simulink model "Molehill"  (Simulink 8.5)
settings: Solver=ode3  StartTime=0.0  StopTime=inf  FixedStep=0.001  RelTol=1e-3
undefined symbols (not defined in the file or in its folder): seedc, seedn
libraries: slrtlib x7, xpcquanserlib x4
settings Model: Creator=Ninad  LastModifiedBy=Ryan  SimulationMode=external
settings SolverCC: EnableConcurrentExecution=on
settings OptimizationCC: BlockReduction=off  OptimizeBlockIOStorage=off  BufferReuse=off  GlobalBufferReuse=off  ExpressionFolding=off  LocalBlockOutputs=off
settings DebuggingCC: SolverPrmCheckMsg=warning  FcnCallInpInsideContextMsg=UseLocalSettings
settings HardwareCC: ProdIntDivRoundTo=Zero  ProdEndianess=LittleEndian  ProdLongLongMode=on  ProdHWDeviceType=Generic->32-bit x86 compatible
settings RTWCC: SystemTargetFile=slrt.tlc  TemplateMakefile=slrt_default_tmf  Description=Simulink Real-Time  RTWCompilerOptimization=on
settings SimulinkRealTimeCC: GeneratePreprocessorConditionals=Disable all

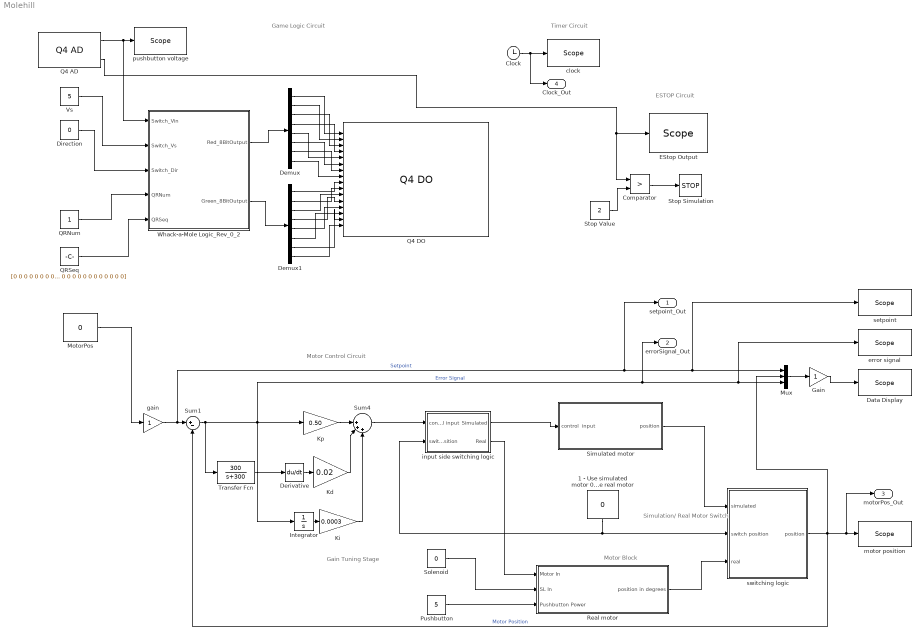
== system Molehill ==
  note: Gain Tuning Stage
  note: Motor Control Circuit
  note: Simulation/
      | Real Motor
      | Switch
  note: Game Logic Circuit
  note: ESTOP Circuit
  note: Timer Circuit
  note: Motor Block
  1 - Use simulated motor 0 - Use real motor : Constant  Value=0
  Clock : Clock
  Comparator : RelationalOperator  Operator=>  OutDataTypeStr=boolean
  Data Display : slrtlib/Displays and Logging/Scope   scopeno=3  scopetype=Target  autostart=on  viewmode=Numerical  formatstr="'Setpoint        %3.2f,Motor Position  %3.2f,Error Signal    %3.2f'"  grid=on  ylimits=[0,170]  nosamples=200  noprepostsamples=0  interleave=10  triggermode=FreeRun  triggersignal=1  trigsignalfromport=off  triggerlevel=0.0  triggerslope=Either  triggerscope=1  triggersample=0  filename=data.dat  mode=Lazy  writesize=512  autorestart=off  dynamicfilemode=off  maxwritefilesize=512*1024^2
  Demux : Demux  Outputs=8
  Demux1 : Demux  Outputs=8
  Derivative : Derivative
  Direction : Constant  Value=0
  "EStop Output " : slrtlib/Displays and Logging/Scope   scopeno=6  scopetype=Target  autostart=on  viewmode=Graphical redraw  formatstr='%15.6f'  grid=on  ylimits=[-6,6]  nosamples=250  noprepostsamples=0  interleave=1  triggermode=FreeRun  triggersignal=1  trigsignalfromport=off  triggerlevel=0.0  triggerslope=Either  triggerscope=1  triggersample=0  filename=data.dat  mode=Lazy  writesize=512  autorestart=off  dynamicfilemode=off  maxwritefilesize=512*1024^2
  Gain : Gain
  Integrator : Integrator
  Kd : Gain  Gain=0.02
  Ki : Gain  Gain=0.0003
  Kp : Gain  Gain=0.50
  MotorPos : Constant  Value=0
  Mux : Mux  Inputs=3
  Pushbutton : Constant  Value=5
  Q4 AD : xpcquanserlib/A//D/Q4 AD  channel=[3 4]  sampleTime=0.001  slot=-1
  "Q4 DO " : xpcquanserlib/Digital Output/Q4 DO   channel=[1 2 3 4 5 6 7 8 9 10 11 12 13 14 15 16]  reset=[1]  initValue=[0 0 0 0 0 0 0 0 0 0 0 0 0 0 0 0]  sampleTime=.001  slot=-1
  QRNum : Constant
  QRSeq : Constant  Value=[0 0 0 0 0 0 0 0 0 0 0 0 0 0 0 0 0 0 0 0]
  Real motor : Subsystem
  Simulated motor : Subsystem
  Solenoid : Constant  Value=0
  Stop Simulation : Stop
  Stop Value : Constant  Value=2
  Sum1 : Sum  Inputs=|+-
  Sum4 : Sum  Inputs=||+++
  Transfer Fcn : TransferFcn  Numerator=[300]  Denominator=[1 300]
  Vs : Constant  Value=5
  Whack-a-Mole Logic_Rev_0_2 : Subsystem  StartFcn=|
      | seedc=seedc+1;
      | seedn=seedn+1;
  clock : slrtlib/Displays and Logging/Scope   scopeno=5  scopetype=Target  autostart=on  viewmode=Numerical  formatstr='%1.3f'  grid=on  ylimits=[-0.2, 1.2]  nosamples=250  noprepostsamples=0  interleave=1  triggermode=FreeRun  triggersignal=1  trigsignalfromport=off  triggerlevel=0.0  triggerslope=Either  triggerscope=1  triggersample=0  filename=data.dat  mode=Lazy  writesize=512  autorestart=off  dynamicfilemode=off  maxwritefilesize=512*1024^2
  error signal : slrtlib/Displays and Logging/Scope   scopeno=2  scopetype=Target  autostart=on  viewmode=Graphical rolling  formatstr='%15.6f'  grid=on  ylimits=[-180,180]  nosamples=500  noprepostsamples=0  interleave=10  triggermode=FreeRun  triggersignal=1  trigsignalfromport=off  triggerlevel=0.0  triggerslope=Either  triggerscope=1  triggersample=0  filename=data.dat  mode=Lazy  writesize=512  autorestart=off  dynamicfilemode=off  maxwritefilesize=512*1024^2
  gain : Gain
  input side switching logic : Subsystem
  motor position : slrtlib/Displays and Logging/Scope   scopeno=7  scopetype=Target  autostart=on  viewmode=Graphical rolling  formatstr='%15.6f'  grid=on  ylimits=[-180,180]  nosamples=500  noprepostsamples=0  interleave=10  triggermode=FreeRun  triggersignal=1  trigsignalfromport=off  triggerlevel=0.0  triggerslope=Either  triggerscope=1  triggersample=0  filename=data.dat  mode=Lazy  writesize=512  autorestart=off  dynamicfilemode=off  maxwritefilesize=512*1024^2
  "pushbutton voltage " : slrtlib/Displays and Logging/Scope   scopeno=4  scopetype=Target  autostart=on  viewmode=Numerical  formatstr='%1.3f'  grid=on  ylimits=[-0.2, 1.2]  nosamples=250  noprepostsamples=0  interleave=1  triggermode=FreeRun  triggersignal=1  trigsignalfromport=off  triggerlevel=0.0  triggerslope=Either  triggerscope=1  triggersample=0  filename=data.dat  mode=Lazy  writesize=512  autorestart=off  dynamicfilemode=off  maxwritefilesize=512*1024^2
  setpoint : slrtlib/Displays and Logging/Scope   scopeno=1  scopetype=Target  autostart=on  viewmode=Graphical rolling  formatstr='%15.6f'  grid=on  ylimits=[-180,180]  nosamples=500  noprepostsamples=0  interleave=10  triggermode=FreeRun  triggersignal=1  trigsignalfromport=off  triggerlevel=0.0  triggerslope=Either  triggerscope=1  triggersample=0  filename=data.dat  mode=Lazy  writesize=512  autorestart=off  dynamicfilemode=off  maxwritefilesize=512*1024^2
  switching logic : Subsystem
  setpoint_Out : Outport
  errorSignal_Out : Outport  Port=2
  motorPos_Out : Outport  Port=3
  Clock_Out : Outport  Port=4
  wires:
  Kp/1 -> Sum4/1
  Kd/1 -> Sum4/2
  Derivative/1 -> Kd/1
  Integrator/1 -> Ki/1
  Ki/1 -> Sum4/3
  gain/1 -> Sum1/1, Mux/1, setpoint/1, setpoint_Out/1  "Setpoint"
  MotorPos/1 -> gain/1
  input side switching logic/1(Simulated) -> Simulated motor/1(control  input)
  input side switching logic/2(Real) -> Real motor/1(Motor In)
  Simulated motor/1(position) -> switching logic/1(simulated)
  Real motor/1(position in degrees) -> switching logic/3(real)
  switching logic/1(position) -> Mux/2, Sum1/2, motor position/1, motorPos_Out/1  "Motor Position"
  Sum4/1 -> input side switching logic/1(control input)
  1 - Use simulated motor 0 - Use real motor/1 -> switching logic/2(switch position), input side switching logic/2(switch  position)
  Gain/1 -> Data Display/1
  Mux/1 -> Gain/1
  Sum1/1 -> Mux/3, error signal/1, errorSignal_Out/1, Kp/1, Integrator/1, Transfer Fcn/1  "Error Signal"
  Comparator/1 -> Stop Simulation/1
  Stop Value/1 -> Comparator/2
  Q4 AD/2 -> Comparator/1, "EStop Output "/1
  Clock/1 -> Clock_Out/1, clock/1
  Whack-a-Mole Logic_Rev_0_2/1(Red_8BitOutput) -> Demux/1
  Whack-a-Mole Logic_Rev_0_2/2(Green_8BitOutput) -> Demux1/1
  Direction/1 -> Whack-a-Mole Logic_Rev_0_2/3(Switch_Dir)
  Vs/1 -> Whack-a-Mole Logic_Rev_0_2/2(Switch_Vs)
  QRNum/1 -> Whack-a-Mole Logic_Rev_0_2/4(QRNum)
  QRSeq/1 -> Whack-a-Mole Logic_Rev_0_2/5(QRSeq)
  Q4 AD/1 -> Whack-a-Mole Logic_Rev_0_2/1(Switch_Vin), "pushbutton voltage "/1
  Demux/8 -> "Q4 DO "/8
  Demux/7 -> "Q4 DO "/7
  Demux/6 -> "Q4 DO "/6
  Demux/5 -> "Q4 DO "/5
  Demux/4 -> "Q4 DO "/4
  Demux/3 -> "Q4 DO "/3
  Demux/2 -> "Q4 DO "/2
  Demux/1 -> "Q4 DO "/1
  Demux1/1 -> "Q4 DO "/9
  Demux1/2 -> "Q4 DO "/10
  Demux1/3 -> "Q4 DO "/11
  Demux1/4 -> "Q4 DO "/12
  Demux1/5 -> "Q4 DO "/13
  Demux1/6 -> "Q4 DO "/14
  Demux1/7 -> "Q4 DO "/15
  Demux1/8 -> "Q4 DO "/16
  Transfer Fcn/1 -> Derivative/1
  Solenoid/1 -> Real motor/2(SL In)
  Pushbutton/1 -> Real motor/3(Pushbutton Power)

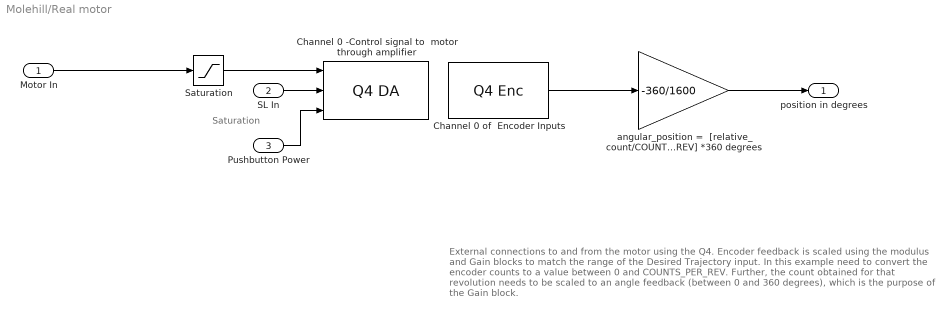
== system Molehill/Real motor ==
  note: Saturation
  note: External connections to and from the motor using the Q4.
      |
      | Encoder feedback is scaled using the modulus and Gain blocks to
      | match the range of the Desired Trajectory input.
      |
      | In this example need to convert the encoder counts to a value between 0 and COUNTS_PER_REV.
      | Further, the count obtained for that revolution needs to be scaled to an angle feedback (between
      | 0 and 360 degrees), which is the purpose of the Gain block.
  Motor In : Inport
  SL In : Inport  Port=2
  Pushbutton Power : Inport  Port=3
  "Channel 0 -Control signal to  motor through amplifier " : xpcquanserlib/D//A/Q4 DA   channel=[1 2 3]  range=[-10]  simul=off  reset=[1]  initValue=[0 0 0]  sampleTime=.001  slot=-1
  "Channel 0 of  Encoder Inputs " : xpcquanserlib/Incremental Encoder/Q4 Enc   channel=[1]  initialCount=[0]  prescale=[1]  quadrature=[4]  mode=[0]  synchronousIndex=[0]  indexPolarity=[0]  preserveCounts=[0]  sampleTime=.001  slot=-1
  Saturation : Saturate  UpperLimit=10  LowerLimit=-10
  angular_position =  [relative_count/COUNTS_PER_REV] *360 degrees : Gain  Gain=-360/1600
  position in degrees : Outport
  wires:
  Saturation/1 -> "Channel 0 -Control signal to  motor through amplifier "/1
  angular_position =  [relative_count/COUNTS_PER_REV] *360 degrees/1 -> position in degrees/1
  "Channel 0 of  Encoder Inputs "/1 -> angular_position =  [relative_count/COUNTS_PER_REV] *360 degrees/1
  Motor In/1 -> Saturation/1
  SL In/1 -> "Channel 0 -Control signal to  motor through amplifier "/2
  Pushbutton Power/1 -> "Channel 0 -Control signal to  motor through amplifier "/3

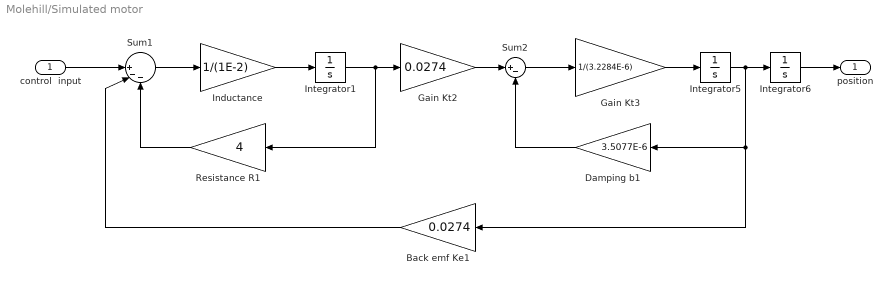
== system Molehill/Simulated motor ==
  control  input : Inport
  Back emf Ke1 : Gain  Gain=0.0274
  Damping b1 : Gain  Gain=3.5077E-6
  Gain Kt2 : Gain  Gain=0.0274
  Gain Kt3 : Gain  Gain=1/(3.2284E-6)
  Inductance : Gain  Gain=1/(1E-2)
  Integrator1 : Integrator
  Integrator5 : Integrator
  Integrator6 : Integrator
  Resistance R1 : Gain  Gain=4
  Sum1 : Sum  Inputs=||+--
  Sum2 : Sum  Inputs=|+-
  position : Outport
  wires:
  Sum1/1 -> Inductance/1
  Inductance/1 -> Integrator1/1
  Integrator1/1 -> Gain Kt2/1, Resistance R1/1
  Gain Kt2/1 -> Sum2/1
  Sum2/1 -> Gain Kt3/1
  Gain Kt3/1 -> Integrator5/1
  Integrator5/1 -> Integrator6/1, Back emf Ke1/1, Damping b1/1
  Back emf Ke1/1 -> Sum1/2
  Damping b1/1 -> Sum2/2
  Resistance R1/1 -> Sum1/3
  Integrator6/1 -> position/1
  control  input/1 -> Sum1/1

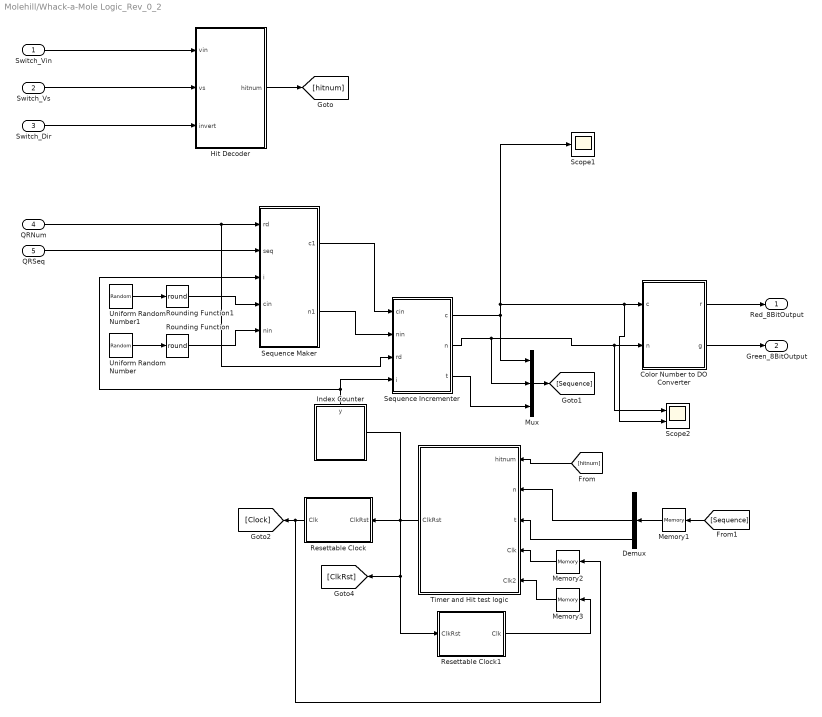
== system Molehill/Whack-a-Mole Logic_Rev_0_2 ==
  Switch_Vin : Inport
  Switch_Vs : Inport  Port=2
  Switch_Dir : Inport  Port=3
  QRNum : Inport  Port=4
  QRSeq : Inport  Port=5
  Color Number to DO Converter : MATLAB Function  TreatAsAtomicUnit=on
  Demux : Demux  Outputs=3
  Hit Decoder : MATLAB Function  TreatAsAtomicUnit=on
  Index Counter : Stateflow chart  TreatAsAtomicUnit=on
  Memory1 : Memory
  Memory2 : Memory
  Memory3 : Memory
  Mux : Mux  Inputs=3
  Resettable Clock : Subsystem
  Resettable Clock1 : Subsystem
  Rounding Function : Rounding  Operator=round
  Rounding Function1 : Rounding  Operator=round
  Scope1 : Scope  NumInputPorts=3
      settings: TimeRange=96.38  YMin=-1~0~-1  YMax=1~4~1
  Scope2 : Scope  NumInputPorts=2
      settings: YMin=0~0  YMax=7~3  SaveName=ScopeData2
  Sequence Incrementer : MATLAB Function  TreatAsAtomicUnit=on
  Sequence Maker : MATLAB Function  TreatAsAtomicUnit=on
  Timer and Hit test logic : Stateflow chart  TreatAsAtomicUnit=on
  Uniform Random Number : UniformRandomNumber  Minimum=0.51  Maximum=8.49  Seed=seedn
  Uniform Random Number1 : UniformRandomNumber  Minimum=0.51  Maximum=3.49  Seed=seedc
  Red_8BitOutput : Outport
  Green_8BitOutput : Outport  Port=2
  wires:
  Resettable Clock1/1(Clk) -> Memory3/1
  Memory3/1 -> Timer and Hit test logic/5(Clk2)
  Uniform Random Number/1 -> Rounding Function/1
  Uniform Random Number1/1 -> Rounding Function1/1
  Hit Decoder/1(hitnum) -> [hitnum]
  Switch_Vs/1 -> Hit Decoder/2(vs)
  Switch_Vin/1 -> Hit Decoder/1(vin)
  Switch_Dir/1 -> Hit Decoder/3(invert)
  Color Number to DO Converter/1(r) -> Red_8BitOutput/1
  Color Number to DO Converter/2(g) -> Green_8BitOutput/1
  Timer and Hit test logic/1(ClkRst) -> [ClkRst], Resettable Clock1/1(ClkRst), Resettable Clock/1(ClkRst), Index Counter/Trigger
  QRSeq/1 -> Sequence Maker/2(seq)
  QRNum/1 -> Sequence Maker/1(rd), Sequence Incrementer/3(rd)
  Index Counter/1(y) -> Sequence Incrementer/4(i), Sequence Maker/3(i)
  Sequence Incrementer/2(n) -> Color Number to DO Converter/2(n), Scope2/1, Mux/2
  Sequence Incrementer/1(c) -> Color Number to DO Converter/1(c), Scope2/2, Scope1/2, Mux/1
  Sequence Incrementer/3(t) -> Mux/3
  [hitnum] -> Timer and Hit test logic/1(hitnum)
  Mux/1 -> [Sequence]
  Memory2/1 -> Timer and Hit test logic/4(Clk)
  Resettable Clock/1(Clk) -> Memory2/1, [Clock]
  [Sequence] -> Memory1/1
  Memory1/1 -> Demux/1
  Rounding Function1/1 -> Sequence Maker/4(cin)
  Rounding Function/1 -> Sequence Maker/5(nin)
  Demux/3 -> Timer and Hit test logic/3(t)
  Demux/2 -> Timer and Hit test logic/2(n)
  Sequence Maker/1(c1) -> Sequence Incrementer/1(cin)
  Sequence Maker/2(n1) -> Sequence Incrementer/2(nin)

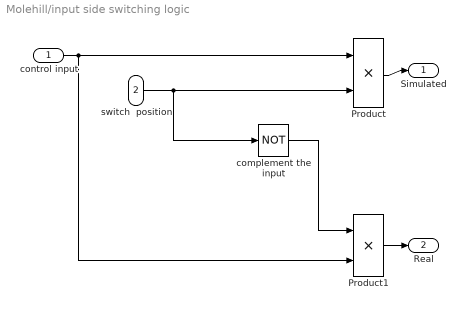
== system Molehill/input side switching logic ==
  control input : Inport
  switch  position : Inport  Port=2
  Product : Product  RndMeth=Zero
  Product1 : Product  RndMeth=Zero
  complement the input : Logic  Operator=NOT  AllPortsSameDT=off  OutDataTypeStr=boolean
  Simulated : Outport
  Real : Outport  Port=2
  wires:
  control input/1 -> Product/1, Product1/2
  complement the input/1 -> Product1/1
  switch  position/1 -> Product/2, complement the input/1
  Product/1 -> Simulated/1
  Product1/1 -> Real/1

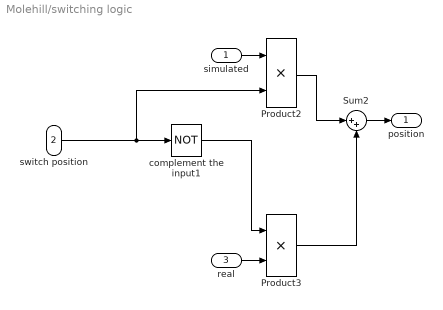
== system Molehill/switching logic ==
  simulated : Inport
  switch position : Inport  Port=2
  real : Inport  Port=3
  Product2 : Product  RndMeth=Zero
  Product3 : Product  RndMeth=Zero
  Sum2 : Sum  Inputs=|++
  complement the input1 : Logic  Operator=NOT  AllPortsSameDT=off  OutDataTypeStr=boolean
  position : Outport
  wires:
  complement the input1/1 -> Product3/1
  Product2/1 -> Sum2/1
  Product3/1 -> Sum2/2
  switch position/1 -> Product2/2, complement the input1/1
  simulated/1 -> Product2/1
  Sum2/1 -> position/1
  real/1 -> Product3/2

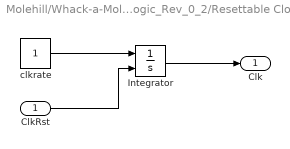
== system Molehill/Whack-a-Mole Logic_Rev_0_2/Resettable Clock ==
  ClkRst : Inport
  Integrator : Integrator  ExternalReset=rising
  clkrate : Constant
  Clk : Outport
  wires:
  clkrate/1 -> Integrator/1
  ClkRst/1 -> Integrator/2
  Integrator/1 -> Clk/1

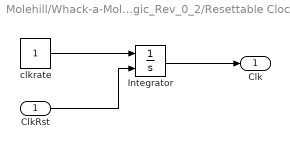
== system Molehill/Whack-a-Mole Logic_Rev_0_2/Resettable Clock1 ==
  ClkRst : Inport
  Integrator : Integrator  ExternalReset=rising
  clkrate : Constant
  Clk : Outport
  wires:
  Integrator/1 -> Clk/1
  ClkRst/1 -> Integrator/2
  clkrate/1 -> Integrator/1

== matlab function Whack-a-Mole Logic_Rev_0_2/Color Number to DO Converter ==
  data: c input double; r output double; n input double; g output double
function [r,g] = fcn(c,n)
% LED Output Block 1.0 - HDK
% This block outputs two 8 bit outputs, one for red LEDs, one for green LEDs. 

% INPUTS
% c     = Color - 1=red, 2=green
% n     = Number - 1-8

% OUTPUTS
% r     = Red outputs 1-8
% g     = Green outputs 1-8

% Outputs are 8 binary values based on what c and n are.

r=zeros(8,1);
g=zeros(8,1);
r=(c==1 || c==3)*[(n==1);(n==2);(n==3);(n==4);(n==5);(n==6);(n==7);(n==8)];
g=(c==2 || c==3)*[(n==1);(n==2);(n==3);(n==4);(n==5);(n==6);(n==7);(n==8)];
end

== matlab function Whack-a-Mole Logic_Rev_0_2/Hit Decoder ==
  data: hitnum output double; vin input double; vs input double; invert input double
function hitnum  = fcn(vin,vs,invert)
% Hit Decoder Block Version 1.0 - HDK
% This block decodes which button is pressed. 

% INPUTS
% Vin       = measured voltage on analogue in.
% Vs        = supply voltage to the switches.
% invert    = Set to 1 if switch order is reversed.

% OUTPUTS
% hitnum    = Pressed button number.

% Voltage levels are normalized by supply voltage.
% MODIFY THESE NUMBERS AT YOUR OWN RISK.

vin2=vin/vs;
if (invert==0)                          % Forward Switch Order
    if (vin2>0.1 && vin2<0.15)
        hitnum=1;
    elseif (vin2>0.225 && vin2<0.275)
        hitnum=2;
	elseif (vin2>0.350 && vin2<0.400)
        hitnum=3;
	elseif (vin2>0.475 && vin2<0.525)
        hitnum=4;
	elseif (vin2>0.600 && vin2<0.650)
        hitnum=5;
	elseif (vin2>0.725 && vin2<0.775)
        hitnum=6;
	elseif (vin2>0.850 && vin2<0.900)
        hitnum=7;
	elseif (vin2>0.975 && vin2<1.025)
        hitnum=8;        
    else
        hitnum=0;
    end
else                                    % Inverted Switch Order
    if (vin2>0.1 && vin2<0.15)
        hitnum=8;
    elseif (vin2>0.225 && vin2<0.275)
        hitnum=7;
	elseif (vin2>0.350 && vin2<0.400)
        hitnum=6;
	elseif (vin2>0.475 && vin2<0.525)
        hitnum=5;
	elseif (vin2>0.600 && vin2<0.650)
        hitnum=4;
	elseif (vin2>0.725 && vin2<0.775)
        hitnum=3;
	elseif (vin2>0.850 && vin2<0.900)
        hitnum=2;
	elseif (vin2>0.975 && vin2<1.025)
        hitnum=1;        
    else
        hitnum=0;
    end
end  
end

== stateflow chart Whack-a-Mole Logic_Rev_0_2/Index Counter ==
  (default) -> (junction 23) : {y++;}
  data: y output double =1
  events: event input RISING_EDGE_EVENT

== matlab function Whack-a-Mole Logic_Rev_0_2/Sequence Incrementer ==
  data: cin input double; nin input double; rd input double; c output double; n output double; i input double; t output double
function [c,n,t] = fcn(cin,nin,rd,i)
% LED Chart Block Version 2.0 - HDK
% This block decodes which button is pressed. 

% INPUTS
% cin   = Color in
% nin   = Location in
% rd    = Round Number
% i     = Output Sequence Index

% OUTPUTS
% c     = Color Out
% n     = Number Out
% t     = Time Limit Out

% The following block sets the time limit for each round. DO NOT MODIFY.

t=60;
switch rd
    case 1
        t = 60;
    case 2
        t = 30;
    case 3
        t = 15;
    case 4
        t = 5;
end

% Output color and location. DO NOT MODIFY.
if (i>0)
    c=cin(i);
    n=nin(i);
else
    c=0;
    n=0;
end
end

== matlab function Whack-a-Mole Logic_Rev_0_2/Sequence Maker ==
  data: rd input double; seq input double; c1 output double; n1 output double; i input double; cin input double; nin input double
function [c1,n1] = fcn(rd,seq,i,cin,nin)
% LED Sequence Type Selector Version 1.0 - HDK
% This block decides what sequence to output based on round number. 

% INPUTS
% rd    = Round and Version Number from QR Code.
% seq   = The to-hit sequence. This is only used for round 1.
% i     = Output Sequence Index.
% cin   = randomly generated color.
% nin   = randomly generated location.

% OUTPUTS
% c1     = Color Sequence
% n1     = Number Sequence

% Generate blank sequence set
persistent c;
persistent n;

if (isempty(c) || isempty(n) || i==1)
    c=zeros(100,1);
    n=zeros(100,1);
else
end

if (rd==1)                          % For round 1, use seq
    c(1:(length(seq)/2),1)=seq((2*[1:(length(seq)/2)])-1);
    n(1:(length(seq)/2),1)=seq(2*[1:(length(seq)/2)]);          
else                                % For round not 1, add a random value to the end of the blank sequence
    if ((c(i,1)==0 && n(i,1)==0) && i>1)
        c(i,1)=cin;
        n(i,1)=nin;
    else
    end
end
c1=c;
n1=n;

== stateflow chart Whack-a-Mole Logic_Rev_0_2/Timer and Hit test logic ==
  state Init
    en: send(ClkRst)
  state Increment1
    en: send(ClkRst)
  note: Increment the index 'i' if the correct button is pressed or time limit expires
  (default) -> Init
  Increment1 -> Init : [((hitnum==n)  || Clk>t) && Clk2>0.5]
  Init -> Increment1 : [((hitnum==n)  || Clk>t) && Clk2>0.5]
  data: hitnum input double; n input double; t input double; Clk input double; Clk2 input double
  events: ClkRst output EITHER_EDGE_EVENT
